simulink model "serialtest"  (R2017a)
settings: Solver=ode45  StartTime=0.0  StopTime=15  RelTol=1e-3  EnableMultiTasking=on
libraries: instrumentlib x1
settings Model: Creator=EQUIPO  LastModifiedBy=MarioAndres
settings OptimizationCC: LifeSpan=inf
settings DebuggingCC: SFUnexpectedBacktrackingDiag=warning  SFNoUnconditionalDefaultTransitionDiag=warning  SFExecutionAtInitializationDiag=none
settings GRTTargetCC: TargetLangStandard=C89/C90 (ANSI)  GeneratePreprocessorConditionals=Disable all
settings ConfigComp: CovMetricSettings=dw  CovHtmlReporting=on  CovSaveCumulativeToWorkspaceVar=on  CovSaveSingleToWorkspaceVar=on  CovExternalEMLEnable=off

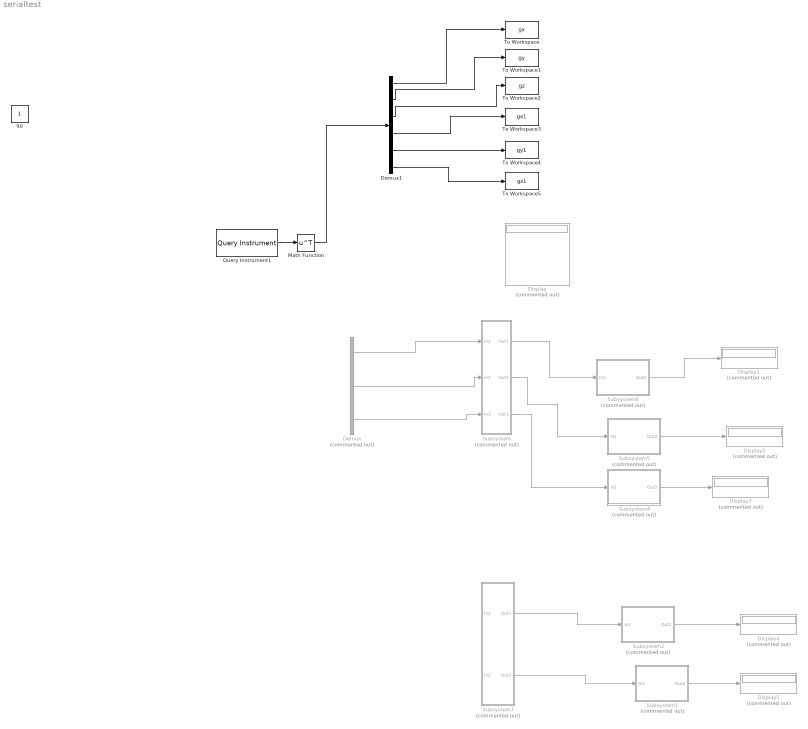
== system serialtest ==
  Demux : Demux  Commented=on  Outputs=3
  Demux1 : Demux  Outputs=6
  Display{,1..5} (6 alike) : Display  Commented=on
  Math Function : Math  Operator=transpose  OutputSignalType=real  SaturateOnIntegerOverflow=on
  Query Instrument1 : instrumentlib/Query Instrument  sampleTime=0.01  isWorkspaceObject=off  timeout=20  inputBufferSize=512  protocol=Serial  serialPort=COM1  baudRate=115200  gpibVendor=Agilent Technologies  boardIndex=0  primaryAddress=1  secondaryAddress=0  visaVendor=Agilent  visaSerialPort=0  chassisIndex=0  logicalAddress=0  tcpRemoteHost='127.0.0.1'  tcpRemotePort=4500  udpRemoteHost='127.0.0.1'  udpRemotePort=9090  visaTCPBoardIndex=0  visaTCPRemoteHost='127.0.0.1'  usbBoardIndex=0  usbManufID=0  usbModelCode=0  usbSerialNumber=0  initAction=None  initCommand='DATA:SOURCE CH1'  initFunction=get  queryCommand='1'  responseFormat=ASCII  asciiFormatting='%d,'  precision=8-bit integer  byteOrder=Little endian  valuesToRead=1  removeBytes=on  afterOutputAction=Repeat query for new data  enableFrames=on  frameSize=6
      settings: SourceProductName=Instrument Control Toolbox  SourceProductBaseCode=IC
  Subsystem : Subsystem  Commented=on
  Subsystem1 : Subsystem  Commented=on
  Subsystem2 : Subsystem  Commented=on
  Subsystem4 : Subsystem  Commented=on
  Subsystem5 : Subsystem  Commented=on
  Subsystem6 : Subsystem  Commented=on
  Subsystem7 : Subsystem  Commented=on
  To Workspace : ToWorkspace  VariableName=gx  SampleTime=0.01
      settings: Save2DSignal=2-D array (concatenate along first dimension)
  To Workspace1 : ToWorkspace  VariableName=gy  SampleTime=0.01
      settings: Save2DSignal=2-D array (concatenate along first dimension)
  To Workspace2 : ToWorkspace  VariableName=gz  SampleTime=0.01
      settings: Save2DSignal=2-D array (concatenate along first dimension)
  To Workspace3 : ToWorkspace  VariableName=gx1  SampleTime=0.01
      settings: Save2DSignal=2-D array (concatenate along first dimension)
  To Workspace4 : ToWorkspace  VariableName=gy1  SampleTime=0.01
      settings: Save2DSignal=2-D array (concatenate along first dimension)
  To Workspace5 : ToWorkspace  VariableName=gz1  SampleTime=0.01
      settings: Save2DSignal=2-D array (concatenate along first dimension)
  90 : Constant  IOType=siggen
  wires:
  Query Instrument1/1 -> Math Function/1
  Math Function/1 -> Demux1/1
  Subsystem2/1(Out2) -> Display4/1
  Subsystem1/1(Out2) -> Display5/1
  Demux/1 -> Subsystem/1(In1)
  Demux/2 -> Subsystem/2(In2)
  Demux/3 -> Subsystem/3(In3)
  Subsystem/1(Out1) -> Subsystem6/1(In1)
  Subsystem/2(Out2) -> Subsystem5/1(In1)
  Subsystem/3(Out3) -> Subsystem4/1(In1)
  Subsystem7/1(Out1) -> Subsystem2/1(In1)
  Subsystem7/2(Out2) -> Subsystem1/1(In1)
  Subsystem5/1(Out2) -> Display2/1
  Subsystem4/1(Out2) -> Display3/1
  Subsystem6/1(Out2) -> Display1/1
  Demux1/1 -> To Workspace/1
  Demux1/2 -> To Workspace1/1
  Demux1/3 -> To Workspace2/1
  Demux1/4 -> To Workspace3/1
  Demux1/5 -> To Workspace4/1
  Demux1/6 -> To Workspace5/1

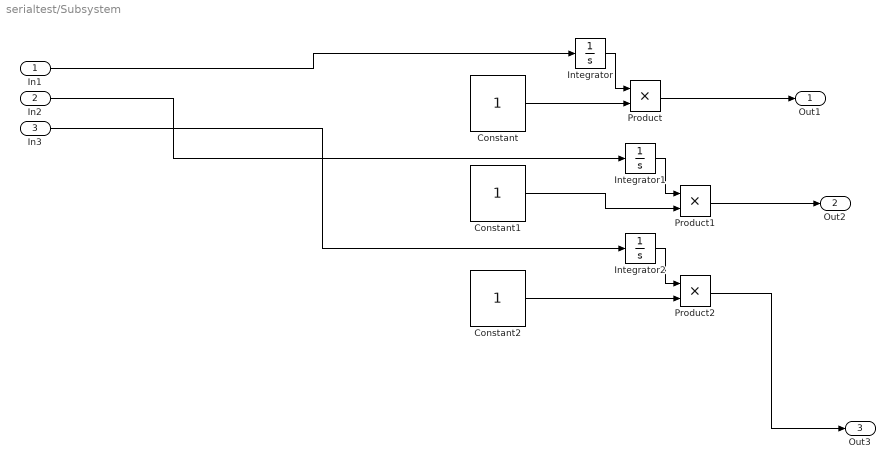
== system serialtest/Subsystem ==
  In1 : Inport
  In2 : Inport  Port=2
  In3 : Inport  Port=3
  Constant : Constant
  Constant1 : Constant
  Constant2 : Constant
  Integrator : Integrator
  Integrator1 : Integrator
  Integrator2 : Integrator
  Product : Product
  Product1 : Product
  Product2 : Product
  Out1 : Outport
  Out2 : Outport  Port=2
  Out3 : Outport  Port=3
  wires:
  In1/1 -> Integrator/1
  In3/1 -> Integrator2/1
  Constant/1 -> Product/2
  Integrator/1 -> Product/1
  Integrator1/1 -> Product1/1
  Constant1/1 -> Product1/2
  In2/1 -> Integrator1/1
  Constant2/1 -> Product2/2
  Integrator2/1 -> Product2/1
  Product/1 -> Out1/1
  Product1/1 -> Out2/1
  Product2/1 -> Out3/1

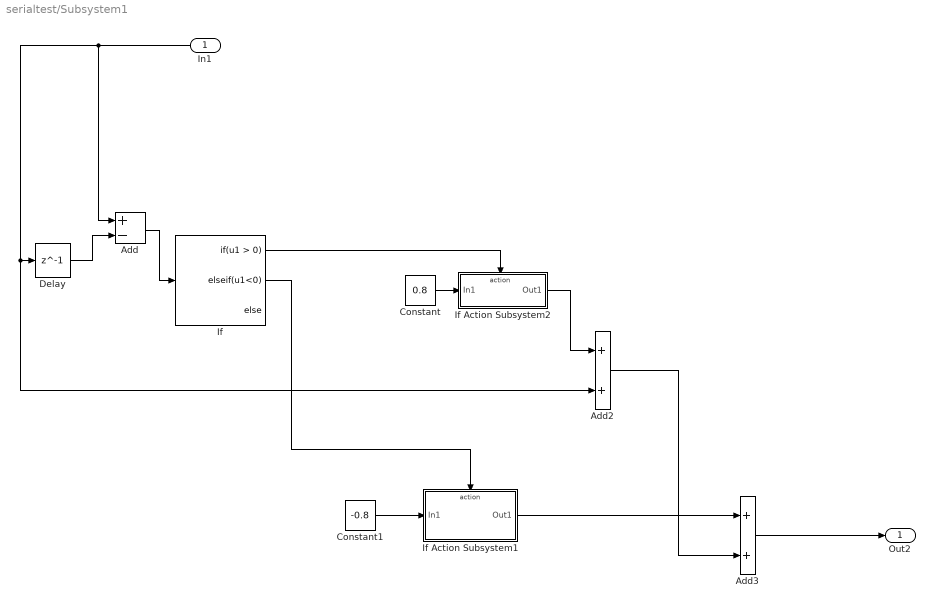
== system serialtest/Subsystem1 ==
  In1 : Inport
  Add : Sum  Inputs=+-
  Add2 : Sum
  Add3 : Sum
  Constant : Constant  Value=0.8
  Constant1 : Constant  Value=-0.8
  Delay : Delay  DelayLength=1  InitialCondition=0  SampleTime=0.01
  If : If  ElseIfExpressions=u1<0
  If Action Subsystem1 : Subsystem  TreatAsAtomicUnit=on
  If Action Subsystem2 : Subsystem  TreatAsAtomicUnit=on
  Out2 : Outport
  wires:
  Delay/1 -> Add/2
  If/1 -> If Action Subsystem2/Action
  Add/1 -> If/1
  If/2 -> If Action Subsystem1/Action
  If Action Subsystem1/1(Out1) -> Add3/1
  Add2/1 -> Add3/2
  Constant1/1 -> If Action Subsystem1/1(In1)
  Add3/1 -> Out2/1
  Constant/1 -> If Action Subsystem2/1(In1)
  If Action Subsystem2/1(Out1) -> Add2/1
  In1/1 -> Add/1, Add2/2, Delay/1

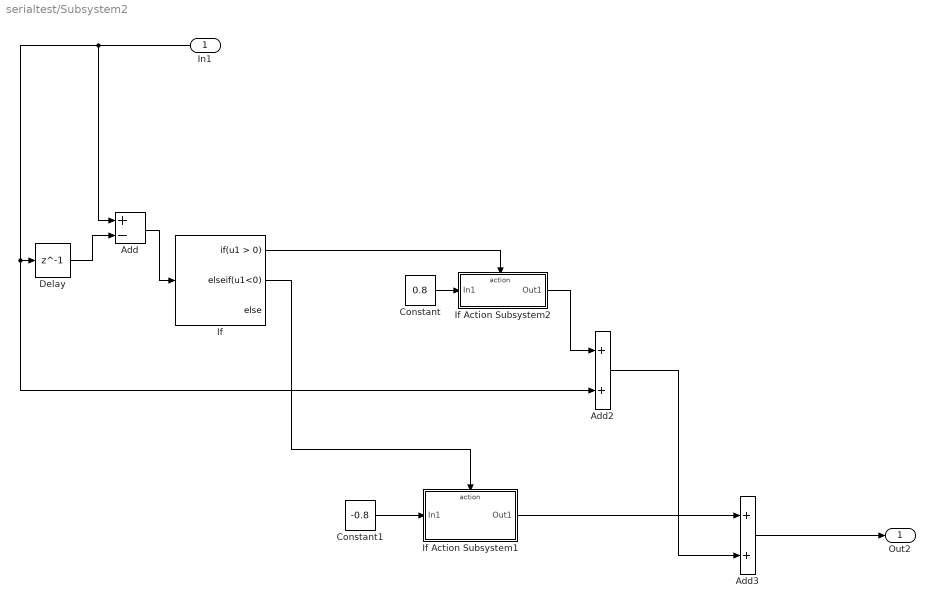
== system serialtest/Subsystem2 ==
  In1 : Inport
  Add : Sum  Inputs=+-
  Add2 : Sum
  Add3 : Sum
  Constant : Constant  Value=0.8
  Constant1 : Constant  Value=-0.8
  Delay : Delay  DelayLength=1  InitialCondition=0  SampleTime=0.01
  If : If  ElseIfExpressions=u1<0
  If Action Subsystem1 : Subsystem  TreatAsAtomicUnit=on
  If Action Subsystem2 : Subsystem  TreatAsAtomicUnit=on
  Out2 : Outport
  wires:
  In1/1 -> Delay/1, Add2/2, Add/1
  If Action Subsystem2/1(Out1) -> Add2/1
  Constant/1 -> If Action Subsystem2/1(In1)
  Add3/1 -> Out2/1
  Constant1/1 -> If Action Subsystem1/1(In1)
  Add2/1 -> Add3/2
  If Action Subsystem1/1(Out1) -> Add3/1
  If/2 -> If Action Subsystem1/Action
  Add/1 -> If/1
  If/1 -> If Action Subsystem2/Action
  Delay/1 -> Add/2

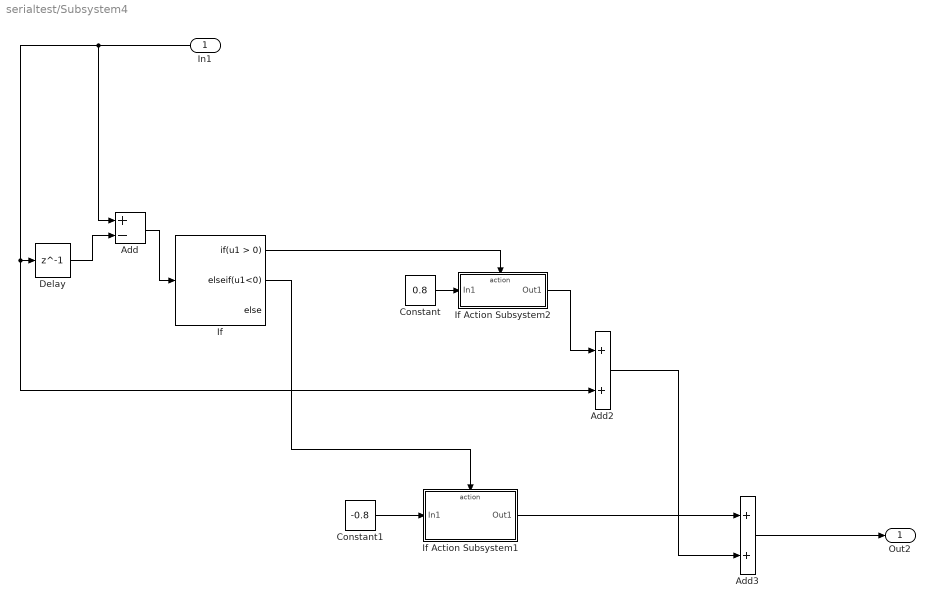
== system serialtest/Subsystem4 ==
  In1 : Inport
  Add : Sum  Inputs=+-
  Add2 : Sum
  Add3 : Sum
  Constant : Constant  Value=0.8
  Constant1 : Constant  Value=-0.8
  Delay : Delay  DelayLength=1  InitialCondition=0  SampleTime=0.005
  If : If  ElseIfExpressions=u1<0
  If Action Subsystem1 : Subsystem  TreatAsAtomicUnit=on
  If Action Subsystem2 : Subsystem  TreatAsAtomicUnit=on
  Out2 : Outport
  wires:
  Delay/1 -> Add/2
  If/1 -> If Action Subsystem2/Action
  Add/1 -> If/1
  If/2 -> If Action Subsystem1/Action
  If Action Subsystem1/1(Out1) -> Add3/1
  Add2/1 -> Add3/2
  Constant1/1 -> If Action Subsystem1/1(In1)
  Add3/1 -> Out2/1
  Constant/1 -> If Action Subsystem2/1(In1)
  If Action Subsystem2/1(Out1) -> Add2/1
  In1/1 -> Add/1, Add2/2, Delay/1

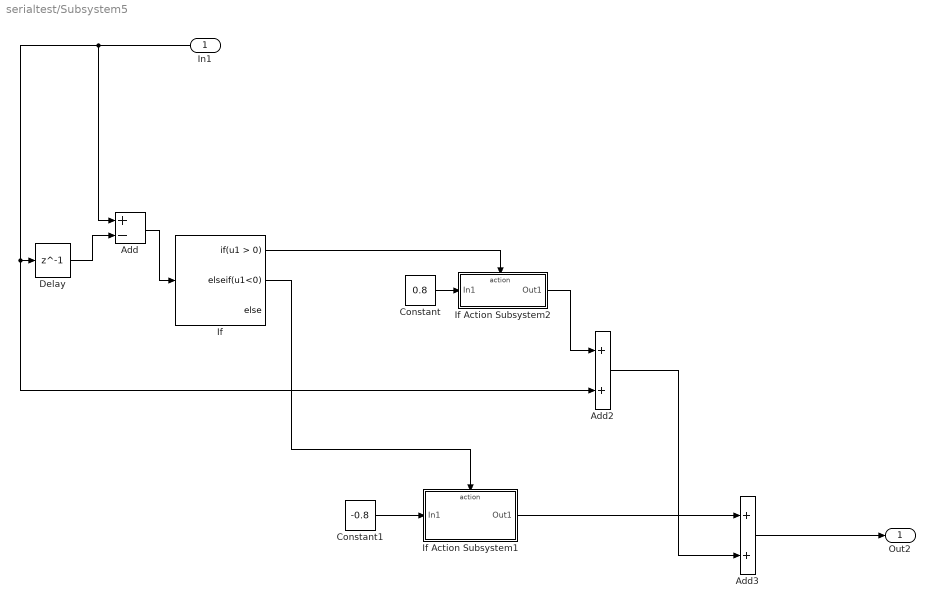
== system serialtest/Subsystem5 ==
  In1 : Inport
  Add : Sum  Inputs=+-
  Add2 : Sum
  Add3 : Sum
  Constant : Constant  Value=0.8
  Constant1 : Constant  Value=-0.8
  Delay : Delay  DelayLength=1  InitialCondition=0  SampleTime=0.005
  If : If  ElseIfExpressions=u1<0
  If Action Subsystem1 : Subsystem  TreatAsAtomicUnit=on
  If Action Subsystem2 : Subsystem  TreatAsAtomicUnit=on
  Out2 : Outport
  wires:
  In1/1 -> Delay/1, Add2/2, Add/1
  If Action Subsystem2/1(Out1) -> Add2/1
  Constant/1 -> If Action Subsystem2/1(In1)
  Add3/1 -> Out2/1
  Constant1/1 -> If Action Subsystem1/1(In1)
  Add2/1 -> Add3/2
  If Action Subsystem1/1(Out1) -> Add3/1
  If/2 -> If Action Subsystem1/Action
  Add/1 -> If/1
  If/1 -> If Action Subsystem2/Action
  Delay/1 -> Add/2

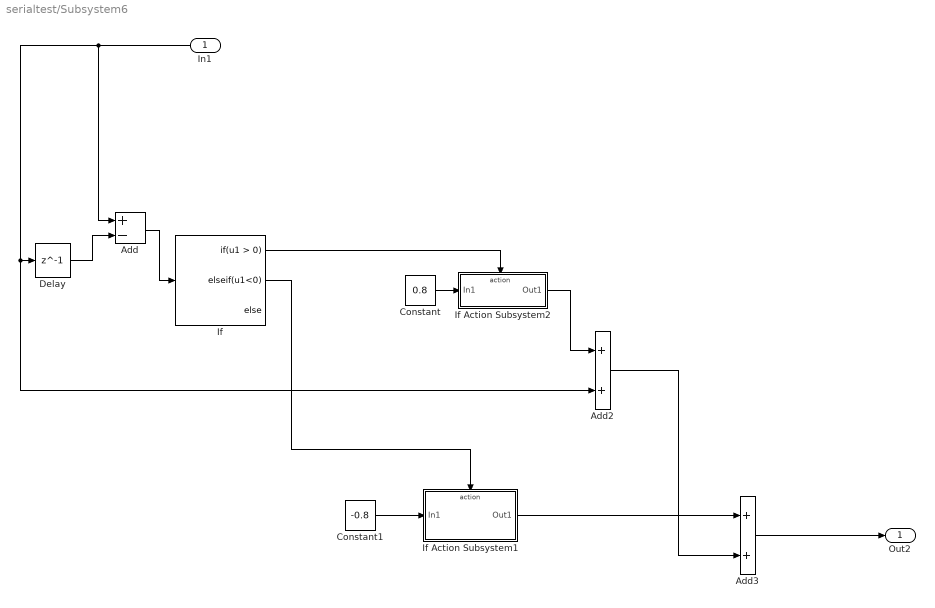
== system serialtest/Subsystem6 ==
  In1 : Inport
  Add : Sum  Inputs=+-
  Add2 : Sum
  Add3 : Sum
  Constant : Constant  Value=0.8
  Constant1 : Constant  Value=-0.8
  Delay : Delay  DelayLength=1  InitialCondition=0  SampleTime=0.005
  If : If  ElseIfExpressions=u1<0
  If Action Subsystem1 : Subsystem  TreatAsAtomicUnit=on
  If Action Subsystem2 : Subsystem  TreatAsAtomicUnit=on
  Out2 : Outport
  wires:
  Delay/1 -> Add/2
  If/1 -> If Action Subsystem2/Action
  Add/1 -> If/1
  If/2 -> If Action Subsystem1/Action
  If Action Subsystem1/1(Out1) -> Add3/1
  Add2/1 -> Add3/2
  Constant1/1 -> If Action Subsystem1/1(In1)
  Add3/1 -> Out2/1
  Constant/1 -> If Action Subsystem2/1(In1)
  If Action Subsystem2/1(Out1) -> Add2/1
  In1/1 -> Add/1, Add2/2, Delay/1

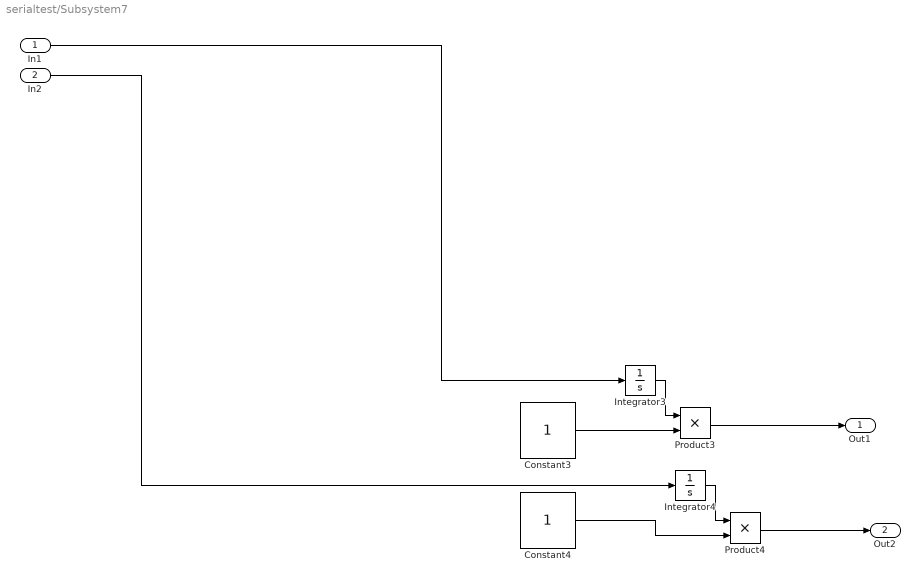
== system serialtest/Subsystem7 ==
  In1 : Inport
  In2 : Inport  Port=2
  Constant3 : Constant
  Constant4 : Constant
  Integrator3 : Integrator
  Integrator4 : Integrator
  Product3 : Product
  Product4 : Product
  Out1 : Outport
  Out2 : Outport  Port=2
  wires:
  Product4/1 -> Out2/1
  Product3/1 -> Out1/1
  In2/1 -> Integrator4/1
  Constant4/1 -> Product4/2
  Integrator4/1 -> Product4/1
  Integrator3/1 -> Product3/1
  Constant3/1 -> Product3/2
  In1/1 -> Integrator3/1

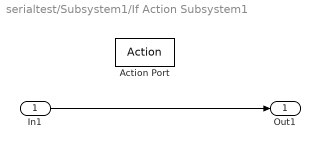
== system serialtest/Subsystem1/If Action Subsystem1 ==
  In1 : Inport
  Action Port : ActionPort  ActionType=elseif
  Out1 : Outport
  wires:
  In1/1 -> Out1/1

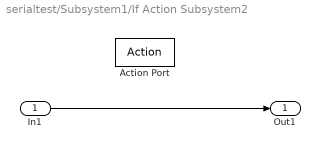
== system serialtest/Subsystem1/If Action Subsystem2 ==
  In1 : Inport
  Action Port : ActionPort  ActionType=then
  Out1 : Outport
  wires:
  In1/1 -> Out1/1

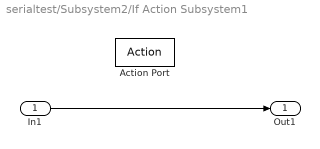
== system serialtest/Subsystem2/If Action Subsystem1 ==
  In1 : Inport
  Action Port : ActionPort  ActionType=elseif
  Out1 : Outport
  wires:
  In1/1 -> Out1/1

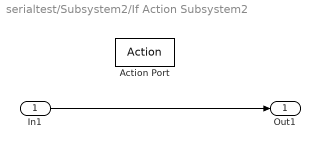
== system serialtest/Subsystem2/If Action Subsystem2 ==
  In1 : Inport
  Action Port : ActionPort  ActionType=then
  Out1 : Outport
  wires:
  In1/1 -> Out1/1

== system serialtest/Subsystem4/If Action Subsystem1 ==
  In1 : Inport
  Action Port : ActionPort  ActionType=elseif
  Out1 : Outport
  wires:
  In1/1 -> Out1/1

== system serialtest/Subsystem4/If Action Subsystem2 ==
  In1 : Inport
  Action Port : ActionPort  ActionType=then
  Out1 : Outport
  wires:
  In1/1 -> Out1/1

== system serialtest/Subsystem5/If Action Subsystem1 ==
  In1 : Inport
  Action Port : ActionPort  ActionType=elseif
  Out1 : Outport
  wires:
  In1/1 -> Out1/1

== system serialtest/Subsystem5/If Action Subsystem2 ==
  In1 : Inport
  Action Port : ActionPort  ActionType=then
  Out1 : Outport
  wires:
  In1/1 -> Out1/1

== system serialtest/Subsystem6/If Action Subsystem1 ==
  In1 : Inport
  Action Port : ActionPort  ActionType=elseif
  Out1 : Outport
  wires:
  In1/1 -> Out1/1

== system serialtest/Subsystem6/If Action Subsystem2 ==
  In1 : Inport
  Action Port : ActionPort  ActionType=then
  Out1 : Outport
  wires:
  In1/1 -> Out1/1
